simulink model "Robust_joint_Space"  (R2020b)
settings: Solver=VariableStepAuto  StartTime=0.0  StopTime=10  RelTol=1e-3
(part 1 of 7)
settings Model: Creator=Ahmadreza  LastModifiedBy=Asus

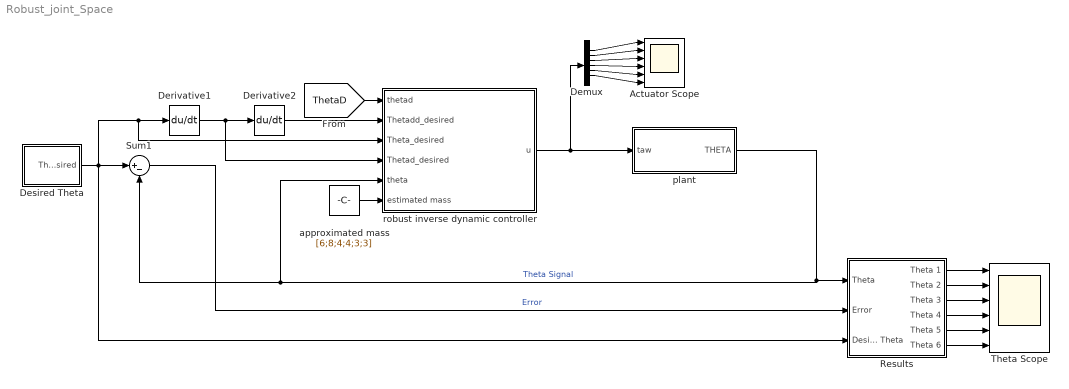
== system Robust_joint_Space ==
  Actuator Scope : Scope  NumInputPorts=6
  Demux : Demux  Outputs=6
  Derivative1 : Derivative
  Derivative2 : Derivative
  Desired Theta : Subsystem
  Results : Subsystem
  Sum1 : Sum  Inputs=|+-
  Theta Scope : Scope  NumInputPorts=6
  approximated mass : Constant  Value=[6;8;4;4;3;3]
  plant : Subsystem
  robust inverse dynamic controller : Subsystem
  wires:
  Derivative1/1 -> robust inverse dynamic controller/4(Thetad_desired), Derivative2/1
  Demux/1 -> Actuator Scope/1
  Demux/2 -> Actuator Scope/2
  Sum1/1 -> Results/2(Error)  "Error"
  Results/4(Theta 4) -> Theta Scope/4
  robust inverse dynamic controller/1(u) -> plant/1(taw), Demux/1
  Demux/6 -> Actuator Scope/6
  Demux/3 -> Actuator Scope/3
  Results/6(Theta 6) -> Theta Scope/6
  Demux/4 -> Actuator Scope/4
  Results/1(Theta 1) -> Theta Scope/1
  Results/2(Theta 2) -> Theta Scope/2
  Results/3(Theta 3) -> Theta Scope/3
  Demux/5 -> Actuator Scope/5
  Desired Theta/1(Theta Desired) -> Results/3(Desired Theta), Derivative1/1, robust inverse dynamic controller/3(Theta_desired), Sum1/1
  Results/5(Theta 5) -> Theta Scope/5
  plant/1(THETA) -> Sum1/2, robust inverse dynamic controller/5(theta), Results/1(Theta)  "Theta Signal"
  approximated mass/1 -> robust inverse dynamic controller/6(estimated mass)
  Derivative2/1 -> robust inverse dynamic controller/2(Thetadd_desired)
  [ThetaD] -> robust inverse dynamic controller/1(thetad)

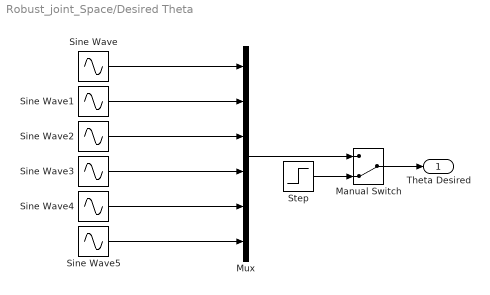
== system Robust_joint_Space/Desired Theta ==
  Manual Switch : ManualSwitch  CurrentSetting=0
  Mux : Mux  Inputs=6
  Sine Wave : Sin  SampleTime=0
  Sine Wave1 : Sin  SampleTime=0
  Sine Wave2 : Sin  SampleTime=0
  Sine Wave3 : Sin  Amplitude=0.5  Bias=0.5  SampleTime=0
  Sine Wave4 : Sin  Amplitude=0.5  Bias=0.5  Frequency=2  SampleTime=0
  Sine Wave5 : Sin  Amplitude=0.5  Bias=0.5  Frequency=0.5  SampleTime=0
  Step : Step  Time=0  Before=[0;0;0;0;0;0];  After=[pi/2;pi/2;pi/2;pi/2;pi/2;pi/2];  SampleTime=0
  Theta Desired : Outport  VectorParamsAs1DForOutWhenUnconnected=off
  wires:
  Sine Wave3/1 -> Mux/4
  Sine Wave/1 -> Mux/1
  Sine Wave2/1 -> Mux/3
  Sine Wave5/1 -> Mux/6
  Sine Wave4/1 -> Mux/5
  Sine Wave1/1 -> Mux/2
  Mux/1 -> Manual Switch/1
  Manual Switch/1 -> Theta Desired/1
  Step/1 -> Manual Switch/2

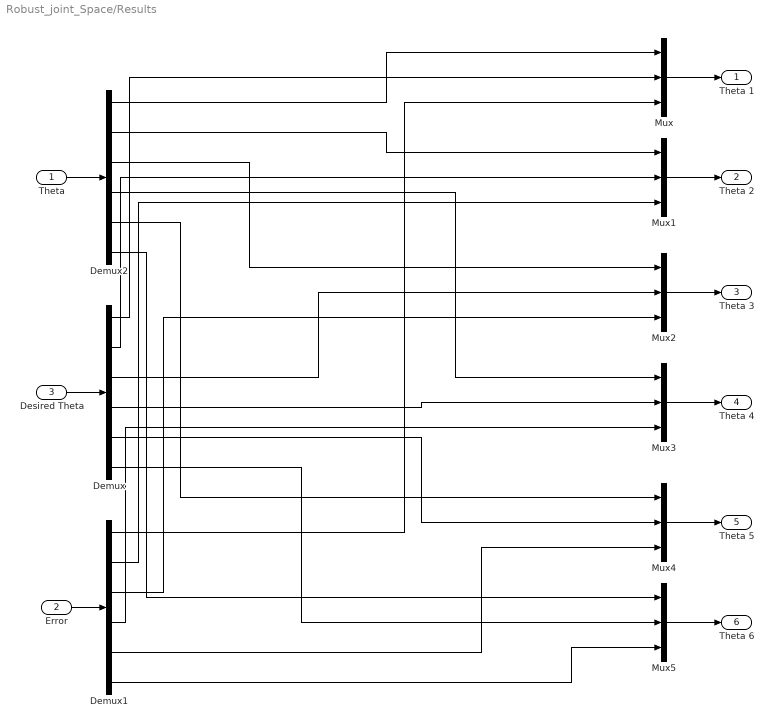
== system Robust_joint_Space/Results ==
  Theta : Inport
  Error : Inport  Port=2
  Desired Theta : Inport  Port=3
  Demux : Demux  Outputs=6
  Demux1 : Demux  Outputs=6
  Demux2 : Demux  Outputs=6
  Mux{,1..5} (6 alike) : Mux  Inputs=3
  Theta 1 : Outport  VectorParamsAs1DForOutWhenUnconnected=off
  Theta 2 : Outport  Port=2  VectorParamsAs1DForOutWhenUnconnected=off
  Theta 3 : Outport  Port=3  VectorParamsAs1DForOutWhenUnconnected=off
  Theta 4 : Outport  Port=4  VectorParamsAs1DForOutWhenUnconnected=off
  Theta 5 : Outport  Port=5  VectorParamsAs1DForOutWhenUnconnected=off
  Theta 6 : Outport  Port=6  VectorParamsAs1DForOutWhenUnconnected=off
  wires:
  Desired Theta/1 -> Demux/1
  Error/1 -> Demux1/1
  Theta/1 -> Demux2/1
  Mux/1 -> Theta 1/1
  Mux1/1 -> Theta 2/1
  Mux2/1 -> Theta 3/1
  Mux3/1 -> Theta 4/1
  Mux4/1 -> Theta 5/1
  Mux5/1 -> Theta 6/1
  Demux2/1 -> Mux/1
  Demux2/2 -> Mux1/1
  Demux2/3 -> Mux2/1
  Demux2/4 -> Mux3/1
  Demux2/5 -> Mux4/1
  Demux2/6 -> Mux5/1
  Demux/1 -> Mux/2
  Demux/2 -> Mux1/2
  Demux/3 -> Mux2/2
  Demux/4 -> Mux3/2
  Demux/5 -> Mux4/2
  Demux/6 -> Mux5/2
  Demux1/1 -> Mux/3
  Demux1/2 -> Mux1/3
  Demux1/3 -> Mux2/3
  Demux1/4 -> Mux3/3
  Demux1/5 -> Mux4/3
  Demux1/6 -> Mux5/3

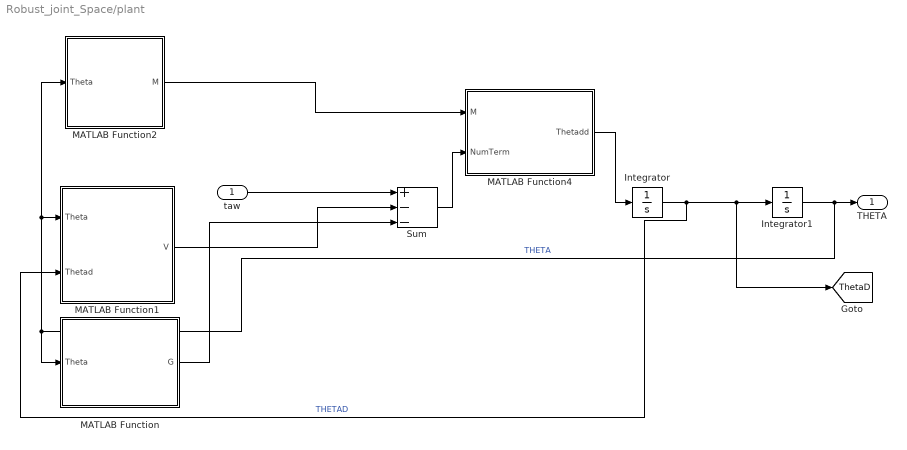
== system Robust_joint_Space/plant ==
  taw : Inport
  Integrator : Integrator  InitialCondition=[0;0;0;0;0;0]
  Integrator1 : Integrator  InitialCondition=[0;0;0;0;0;0]
  MATLAB Function : MATLAB Function  TreatAsAtomicUnit=on
  MATLAB Function1 : MATLAB Function  TreatAsAtomicUnit=on
  MATLAB Function2 : MATLAB Function  TreatAsAtomicUnit=on
  MATLAB Function4 : MATLAB Function  TreatAsAtomicUnit=on
  Sum : Sum  Inputs=+--
  THETA : Outport
  tag scope: ThetaD=global
  wires:
  Integrator/1 -> MATLAB Function1/2(Thetad), [ThetaD], Integrator1/1  "THETAD"
  MATLAB Function4/1(Thetadd) -> Integrator/1
  MATLAB Function1/1(V) -> Sum/2
  MATLAB Function2/1(M) -> MATLAB Function4/1(M)
  Sum/1 -> MATLAB Function4/2(NumTerm)
  Integrator1/1 -> MATLAB Function1/1(Theta), MATLAB Function2/1(Theta), MATLAB Function/1(Theta), THETA/1  "THETA"
  taw/1 -> Sum/1
  MATLAB Function/1(G) -> Sum/3

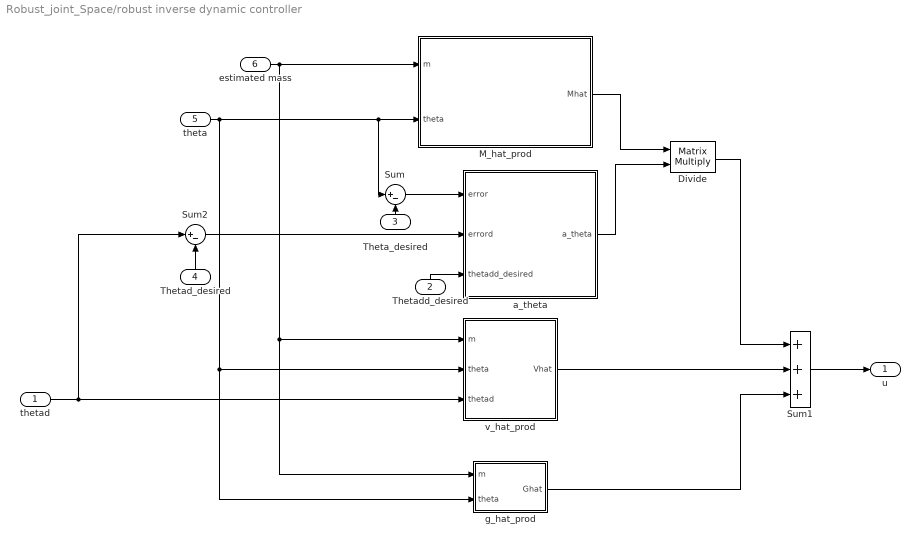
== system Robust_joint_Space/robust inverse dynamic controller ==
  thetad : Inport
  Thetadd_desired : Inport  Port=2
  Theta_desired : Inport  Port=3
  Thetad_desired : Inport  Port=4
  theta : Inport  Port=5
  estimated mass : Inport  Port=6
  Divide : Product  Multiplication=Matrix(*)
  M_hat_prod : MATLAB Function  TreatAsAtomicUnit=on
  Sum : Sum  Inputs=|+-
  Sum1 : Sum  Inputs=+++
  Sum2 : Sum  Inputs=|+-
  a_theta : MATLAB Function  TreatAsAtomicUnit=on
  g_hat_prod : MATLAB Function  TreatAsAtomicUnit=on
  v_hat_prod : MATLAB Function  TreatAsAtomicUnit=on
  u : Outport
  wires:
  a_theta/1(a_theta) -> Divide/2
  Sum1/1 -> u/1
  g_hat_prod/1(Ghat) -> Sum1/3
  Divide/1 -> Sum1/1
  v_hat_prod/1(Vhat) -> Sum1/2
  estimated mass/1 -> M_hat_prod/1(m), v_hat_prod/1(m), g_hat_prod/1(m)
  theta/1 -> g_hat_prod/2(theta), v_hat_prod/2(theta), M_hat_prod/2(theta), Sum/1
  thetad/1 -> v_hat_prod/3(thetad), Sum2/1
  Thetadd_desired/1 -> a_theta/3(thetadd_desired)
  Thetad_desired/1 -> Sum2/2
  Sum2/1 -> a_theta/2(errord)
  Theta_desired/1 -> Sum/2
  Sum/1 -> a_theta/1(error)
  M_hat_prod/1(Mhat) -> Divide/1
